simulink model "AMPC_CSimOldNN_genLinearModelBased"  (R2019b)
settings: Solver=FixedStepAuto  StartTime=0.0  StopTime=Time(end)  FixedStep=Time(2)  RelTol=1e-3
libraries: neural x31, mpclib x1, cstblocks x1
settings Model: Creator=Shouvik Chakraborty  LastModifiedBy=shouv
settings SFSimCC: CustomCodeUndefinedFunction=UseInterfaceOnly

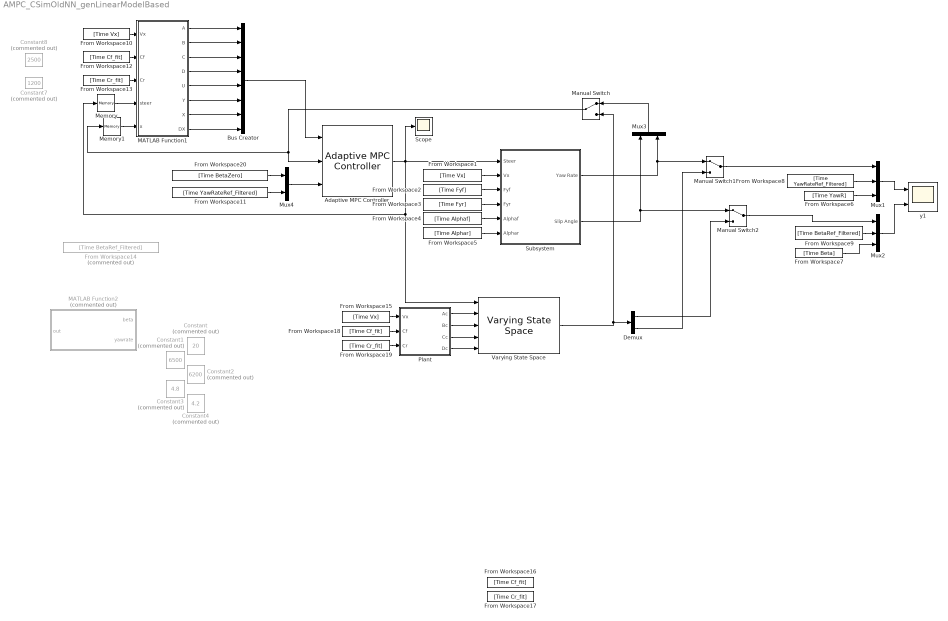
== system AMPC_CSimOldNN_genLinearModelBased ==
  Adaptive MPC Controller : mpclib/Adaptive MPC Controller  SCDEnableBlockLinearizationSpecification=on  mpcobj=adaptivempc1  enable_value=0  updateMPCinCallerWorkspace=on  md_inport=off  mv_inport=off  uref_inport=off  return_cost=off  return_mvseq=off  return_qpstatus=off  return_xseq=off  return_state=off  return_ovseq=off  state_inport=off  isltv_plant=off  umin_inport=off  umax_inport=off  ymin_inport=off  ymax_inport=off  cc_inport=off  ywt_inport=off  uwt_inport=off  duwt_inport=off  rhoeps_inport=off  pm_inport=off  MaximumP=10  HorizonChoice=FixedHorizon  BlockDataType=double  SampleTimeInherited=off  switch_inport=off
      settings: SourceProductName=Model Predictive Control Toolbox
  Bus Creator : BusCreator  Inputs=8
  Constant : Constant  Commented=on  Value=20
  Constant1 : Constant  Commented=on  Value=6500
  Constant2 : Constant  Commented=on  Value=6200
  Constant3 : Constant  Commented=on  Value=4.8
  Constant4 : Constant  Commented=on  Value=4.2
  Constant7 : Constant  Commented=on  Value=1200
  Constant8 : Constant  Commented=on  Value=2500
  Demux : Demux  Outputs=2
  From Workspace1 : FromWorkspace  VariableName=[Time Vx]  SampleTime=0
  From Workspace10 : FromWorkspace  VariableName=[Time Vx]  SampleTime=0
  From Workspace11 : FromWorkspace  VariableName=[Time YawRateRef_Filtered]  SampleTime=0
  From Workspace12 : FromWorkspace  VariableName=[Time Cf_fit]  SampleTime=0
  From Workspace13 : FromWorkspace  VariableName=[Time Cr_fit]  SampleTime=0
  From Workspace14 : FromWorkspace  Commented=on  VariableName=[Time BetaRef_Filtered]  SampleTime=0
  From Workspace15 : FromWorkspace  VariableName=[Time Vx]  SampleTime=0
  From Workspace16 : FromWorkspace  VariableName=[Time Cf_fit]  SampleTime=0
  From Workspace17 : FromWorkspace  VariableName=[Time Cr_fit]  SampleTime=0
  From Workspace18 : FromWorkspace  VariableName=[Time Cf_fit]  SampleTime=0
  From Workspace19 : FromWorkspace  VariableName=[Time Cr_fit]  SampleTime=0
  From Workspace2 : FromWorkspace  VariableName=[Time Fyf]  SampleTime=0
  From Workspace20 : FromWorkspace  VariableName=[Time BetaZero]  SampleTime=0
  From Workspace3 : FromWorkspace  VariableName=[Time Fyr]  SampleTime=0
  From Workspace4 : FromWorkspace  VariableName=[Time Alphaf]  SampleTime=0
  From Workspace5 : FromWorkspace  VariableName=[Time Alphar]  SampleTime=0
  From Workspace6 : FromWorkspace  VariableName=[Time YawR]  SampleTime=0
  From Workspace7 : FromWorkspace  VariableName=[Time Beta]  SampleTime=0
  From Workspace8 : FromWorkspace  VariableName=[Time YawRateRef_Filtered]  SampleTime=0
  From Workspace9 : FromWorkspace  VariableName=[Time BetaRef_Filtered]  SampleTime=0
  MATLAB Function1 : MATLAB Function  TreatAsAtomicUnit=on
  MATLAB Function2 : MATLAB Function  Commented=on  TreatAsAtomicUnit=on
  Manual Switch : ManualSwitch
  Manual Switch1 : ManualSwitch
  Manual Switch2 : ManualSwitch
  Memory : Memory
  Memory1 : Memory
  Mux1 : Mux  Inputs=3
  Mux2 : Mux  Inputs=3
  Mux3 : Mux  Inputs=2
  Mux4 : Mux  Inputs=2
  Plant : MATLAB Function  TreatAsAtomicUnit=on
  Scope : Scope
  Subsystem : Subsystem
  Varying State Space : cstblocks/Linear Parameter Varying/Varying State Space  x0=0  xNames=''  OutputX=off  OutputDX=off
      settings: SourceProductName=Control System Toolbox
  y1 : Scope  NumInputPorts=2
      mask Display: e = 0.06;c1 = [120 230 180]/255;c2 = ([120 230 180]+0)/(256+128);c3 = ([120 230 180]+128)/(256+128);patch([0 1 1 0],[0 0 1 1],c1);patch([0 1 1 1-e 1-e 0+e],[0 0 1 1-e 0+e 0+e],c2);patch([0 0 1 1-e 0+e 0+e],[0 1 1 1-e 1-e 0+e],c3);plot([0 1 1 0 0],[0 0 1 1 0]);plot([0.15 0.85 0.85 0.15 0.15],[0.5 0.5 0.85 0.85 0.5]);
  wires:
  From Workspace7/1 -> Mux2/3
  Mux2/1 -> y1/2
  MATLAB Function1/3(C) -> Bus Creator/3
  MATLAB Function1/5(U) -> Bus Creator/5
  MATLAB Function1/4(D) -> Bus Creator/4
  Mux1/1 -> y1/1
  MATLAB Function1/6(Y) -> Bus Creator/6
  From Workspace11/1 -> Mux4/2
  Subsystem/1(Yaw Rate) -> Mux3/2, Manual Switch1/1
  MATLAB Function1/2(B) -> Bus Creator/2
  Subsystem/2(Slip Angle) -> Manual Switch2/1, Mux3/1
  From Workspace9/1 -> Mux2/2
  MATLAB Function1/1(A) -> Bus Creator/1
  Mux4/1 -> Adaptive MPC Controller/3
  From Workspace1/1 -> Subsystem/2(Vx)
  MATLAB Function1/7(X) -> Bus Creator/7
  Memory/1 -> MATLAB Function1/4(steer)
  MATLAB Function1/8(DX) -> Bus Creator/8
  Bus Creator/1 -> Adaptive MPC Controller/1
  From Workspace5/1 -> Subsystem/6(Alphar)
  From Workspace20/1 -> Mux4/1
  From Workspace6/1 -> Mux1/3
  From Workspace3/1 -> Subsystem/4(Fyr)
  From Workspace12/1 -> MATLAB Function1/2(Cf)
  From Workspace10/1 -> MATLAB Function1/1(Vx)
  From Workspace13/1 -> MATLAB Function1/3(Cr)
  From Workspace8/1 -> Mux1/2
  Manual Switch/1 -> Memory1/1, Adaptive MPC Controller/2
  From Workspace2/1 -> Subsystem/3(Fyf)
  From Workspace4/1 -> Subsystem/5(Alphaf)
  From Workspace15/1 -> Plant/1(Vx)
  From Workspace18/1 -> Plant/2(Cf)
  From Workspace19/1 -> Plant/3(Cr)
  Adaptive MPC Controller/1 -> Varying State Space/1, Memory/1, Subsystem/1(Steer), Scope/1
  Mux3/1 -> Manual Switch/1
  Manual Switch1/1 -> Mux1/1
  Varying State Space/1 -> Demux/1, Manual Switch/2
  Manual Switch2/1 -> Mux2/1
  Demux/1 -> Manual Switch2/2
  Demux/2 -> Manual Switch1/2
  Plant/1(Ac) -> Varying State Space/2
  Plant/2(Bc) -> Varying State Space/3
  Plant/3(Cc) -> Varying State Space/4
  Plant/4(Dc) -> Varying State Space/5
  Memory1/1 -> MATLAB Function1/5(x)

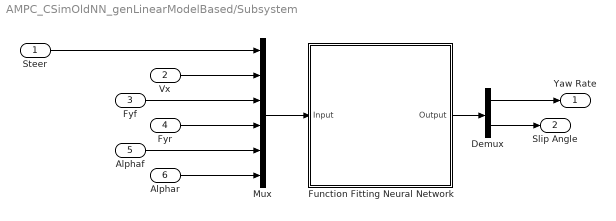
== system AMPC_CSimOldNN_genLinearModelBased/Subsystem ==
  Steer : Inport
  Vx : Inport  Port=2
  Fyf : Inport  Port=3
  Fyr : Inport  Port=4
  Alphaf : Inport  Port=5
  Alphar : Inport  Port=6
  Demux : Demux  Outputs=2
  Function Fitting Neural Network : Subsystem
      mask help: Function Fitting Neural Network
      mask Display: e = 0.06;c1 = [120 150 230]/255;c2 = ([120 150 230]+0)/383;c3 = ([120 150 230]+128)/383;patch([0 1 1 0],[0 0 1 1],c1);patch([0 1 1 1-e 1-e 0+e],[0 0 1 1-e 0+e 0+e],c2);patch([0 0 1 1-e 0+e 0+e],[0 1 1 1-e 1-e 0+e],c3);plot([0 1 1 0 0],[0 0 1 1 0]);fprintf('NNET');port_label('input',1,' Input');port_label('output',1,'Output ');
  Mux : Mux  Inputs=6
  Yaw Rate : Outport  VectorParamsAs1DForOutWhenUnconnected=off
  Slip Angle : Outport  Port=2  VectorParamsAs1DForOutWhenUnconnected=off
  wires:
  Vx/1 -> Mux/2
  Fyr/1 -> Mux/4
  Mux/1 -> Function Fitting Neural Network/1(Input)
  Steer/1 -> Mux/1
  Function Fitting Neural Network/1(Output) -> Demux/1
  Demux/2 -> Slip Angle/1
  Fyf/1 -> Mux/3
  Alphaf/1 -> Mux/5
  Demux/1 -> Yaw Rate/1
  Alphar/1 -> Mux/6

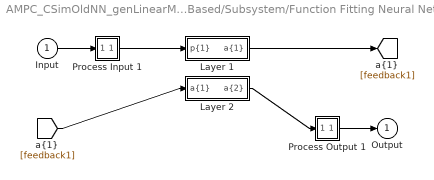
== system AMPC_CSimOldNN_genLinearModelBased/Subsystem/Function Fitting Neural Network ==
  Input : Inport  PortDimensions=6
      mask Display: e = 0.06;c1 = [120 230 180]/255;c2 = ([120 230 180]+0)/(256+128);c3 = ([120 230 180]+128)/(256+128);patch([0 1 1 0],[0 0 1 1],c1);patch([0 1 1 1-e 1-e 0+e],[0 0 1 1-e 0+e 0+e],c2);patch([0 0 1 1-e 0+e 0+e],[0 1 1 1-e 1-e 0+e],c3);plot([0 1 1 0 0],[0 0 1 1 0]);
  Layer 1 : Subsystem
      mask Display: e = 0.06;c1 = [120 150 230]/255;c2 = ([120 150 230]+0)/383;c3 = ([120 150 230]+128)/383;patch([0 1 1 0],[0 0 1 1],c1);patch([0 1 1 1-e 1-e 0+e],[0 0 1 1-e 0+e 0+e],c2);patch([0 0 1 1-e 0+e 0+e],[0 1 1 1-e 1-e 0+e],c3);plot([0 1 1 0 0],[0 0 1 1 0]);
  Layer 2 : Subsystem
      mask Display: e = 0.06;c1 = [120 150 230]/255;c2 = ([120 150 230]+0)/383;c3 = ([120 150 230]+128)/383;patch([0 1 1 0],[0 0 1 1],c1);patch([0 1 1 1-e 1-e 0+e],[0 0 1 1-e 0+e 0+e],c2);patch([0 0 1 1-e 0+e 0+e],[0 1 1 1-e 1-e 0+e],c3);plot([0 1 1 0 0],[0 0 1 1 0]);
  Process Input 1 : Subsystem
      mask Display: e = 0.06;c1 = [120 150 230]/255;c2 = ([120 150 230]+0)/383;c3 = ([120 150 230]+128)/383;patch([0 1 1 0],[0 0 1 1],c1);patch([0 1 1 1-e 1-e 0+e],[0 0 1 1-e 0+e 0+e],c2);patch([0 0 1 1-e 0+e 0+e],[0 1 1 1-e 1-e 0+e],c3);plot([0 1 1 0 0],[0 0 1 1 0]);
  Process Output 1 : Subsystem
      mask Display: e = 0.06;c1 = [120 150 230]/255;c2 = ([120 150 230]+0)/383;c3 = ([120 150 230]+128)/383;patch([0 1 1 0],[0 0 1 1],c1);patch([0 1 1 1-e 1-e 0+e],[0 0 1 1-e 0+e 0+e],c2);patch([0 0 1 1-e 0+e 0+e],[0 1 1 1-e 1-e 0+e],c3);plot([0 1 1 0 0],[0 0 1 1 0]);
  Output : Outport  InitialOutput=[0;0]  VectorParamsAs1DForOutWhenUnconnected=off
      mask Display: e = 0.06;c1 = [120 230 180]/255;c2 = ([120 230 180]+0)/(256+128);c3 = ([120 230 180]+128)/(256+128);patch([0 1 1 0],[0 0 1 1],c1);patch([0 1 1 1-e 1-e 0+e],[0 0 1 1-e 0+e 0+e],c2);patch([0 0 1 1-e 0+e 0+e],[0 1 1 1-e 1-e 0+e],c3);plot([0 1 1 0 0],[0 0 1 1 0]);
  wires:
  Input/1 -> Process Input 1/1(x)
  Process Output 1/1(y) -> Output/1
  Process Input 1/1(p) -> Layer 1/1("p{1}")
  Layer 1/1("a{1}") -> [feedback1]
  [feedback1] -> Layer 2/1("a{1} ")
  Layer 2/1("a{2}") -> Process Output 1/1(a)

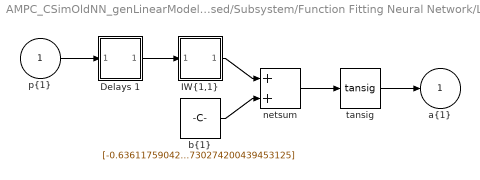
== system AMPC_CSimOldNN_genLinearModelBased/Subsystem/Function Fitting Neural Network/Layer 1 ==
  "p{1}" : Inport  PortDimensions=6
      mask Display: e = 0.06;c1 = [120 230 180]/255;c2 = ([120 230 180]+0)/(256+128);c3 = ([120 230 180]+128)/(256+128);patch([0 1 1 0],[0 0 1 1],c1);patch([0 1 1 1-e 1-e 0+e],[0 0 1 1-e 0+e 0+e],c2);patch([0 0 1 1-e 0+e 0+e],[0 1 1 1-e 1-e 0+e],c3);plot([0 1 1 0 0],[0 0 1 1 0]);
  Delays 1 : Subsystem
      mask Display: e = 0.06;c1 = [120 150 230]/255;c2 = ([120 150 230]+0)/383;c3 = ([120 150 230]+128)/383;patch([0 1 1 0],[0 0 1 1],c1);patch([0 1 1 1-e 1-e 0+e],[0 0 1 1-e 0+e 0+e],c2);patch([0 0 1 1-e 0+e 0+e],[0 1 1 1-e 1-e 0+e],c3);plot([0 1 1 0 0],[0 0 1 1 0]);disp('0');
  "IW{1,1}" : Subsystem
      mask Display: e = 0.06;c1 = [120 150 230]/255;c2 = ([120 150 230]+0)/383;c3 = ([120 150 230]+128)/383;patch([0 1 1 0],[0 0 1 1],c1);patch([0 1 1 1-e 1-e 0+e],[0 0 1 1-e 0+e 0+e],c2);patch([0 0 1 1-e 0+e 0+e],[0 1 1 1-e 1-e 0+e],c3);plot([0 1 1 0 0],[0 0 1 1 0]);disp('W');
  "b{1}" : Constant  Value=[-0.63611759042286653009767860567080788314342498779296875;0.0678442132315502932637940602944581769406795501708984375;0.920857296622486831694232023437507450580596923828125;0.3400400984533717974045430310070514678955078125;1.068840554455138036615835517295636236667633056640625;-1.1840912053117917945854742356459610164165496826171875;2.1641288663140425541087097371928393840789794921875;-0.0026747980112842586163102165386362685239873826503753662109375;-1.2400348389807971383191897984943352639675140380859375;0.05422832279501725583070737002344685606658458709716796875;1.090956117788687063097086138441227376461029052734375;-0.538161801971245079556638302165083587169647216796875;-0.0971368234755809190072994852016563527286052703857421875;-0.65424405420957143508786657548625953495502471923828125;-0.0294578949609712141544104468948717112652957439422607421875;-0.055152953134630144926831007978762499988079071044921875;1.1922936756190452012305058815400116145610809326171875;-0.4982569158340737214274440702865831553936004638671875;1.4572737748217508002568365554907359182834625244140625;-0.71536140771868428345214852015487849712371826171875;0.121920011275389150728898357556317932903766632080078125;-0.08237235483539008529252356538563617505133152008056640625;0.0065354555755173411590863707942844484932720661163330078125;0.57411081788391593594411688172840513288974761962890625;0.890585538278589883276481486973352730274200439453125]
      mask Display: e = 0.06;c1 = [120 150 230]/255;c2 = ([120 150 230]+0)/383;c3 = ([120 150 230]+128)/383;patch([0 1 1 0],[0 0 1 1],c1);patch([0 1 1 1-e 1-e 0+e],[0 0 1 1-e 0+e 0+e],c2);patch([0 0 1 1-e 0+e 0+e],[0 1 1 1-e 1-e 0+e],c3);plot([0 1 1 0 0],[0 0 1 1 0]);disp('b');
  netsum : Sum  Inputs=2  SaturateOnIntegerOverflow=on  InputSameDT=on  OutDataTypeStr=Inherit: Same as first input
      mask Display: e = 0.06;c1 = [120 150 230]/255;c2 = ([120 150 230]+0)/383;c3 = ([120 150 230]+128)/383;patch([0 1 1 0],[0 0 1 1],c1);patch([0 1 1 1-e 1-e 0+e],[0 0 1 1-e 0+e 0+e],c2);patch([0 0 1 1-e 0+e 0+e],[0 1 1 1-e 1-e 0+e],c3);plot([0 1 1 0 0],[0 0 1 1 0]);disp('+');
  tansig : neural/Transfer Functions/tansig
      settings: SourceProductName=MATLAB Runtime - Deep Learning Toolbox  SourceProductBaseCode=Missing
  "a{1}" : Outport  InitialOutput=[0;0;0;0;0;0;0;0;0;0;0;0;0;0;0;0;0;0;0;0;0;0;0;0;0]  VectorParamsAs1DForOutWhenUnconnected=off
      mask Display: e = 0.06;c1 = [120 230 180]/255;c2 = ([120 230 180]+0)/(256+128);c3 = ([120 230 180]+128)/(256+128);patch([0 1 1 0],[0 0 1 1],c1);patch([0 1 1 1-e 1-e 0+e],[0 0 1 1-e 0+e 0+e],c2);patch([0 0 1 1-e 0+e 0+e],[0 1 1 1-e 1-e 0+e],c3);plot([0 1 1 0 0],[0 0 1 1 0]);
  wires:
  "p{1}"/1 -> Delays 1/1("p{1}")
  Delays 1/1("pd{1,1}") -> "IW{1,1}"/1("pd{1,1}")
  "IW{1,1}"/1("iz{1,1}") -> netsum/1
  "b{1}"/1 -> netsum/2
  netsum/1 -> tansig/1
  tansig/1 -> "a{1}"/1

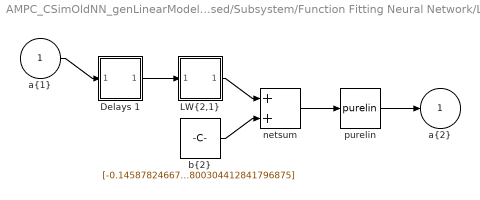
== system AMPC_CSimOldNN_genLinearModelBased/Subsystem/Function Fitting Neural Network/Layer 2 ==
  "a{1} " : Inport  PortDimensions=25
      mask Display: e = 0.06;c1 = [120 230 180]/255;c2 = ([120 230 180]+0)/(256+128);c3 = ([120 230 180]+128)/(256+128);patch([0 1 1 0],[0 0 1 1],c1);patch([0 1 1 1-e 1-e 0+e],[0 0 1 1-e 0+e 0+e],c2);patch([0 0 1 1-e 0+e 0+e],[0 1 1 1-e 1-e 0+e],c3);plot([0 1 1 0 0],[0 0 1 1 0]);
  Delays 1 : Subsystem
      mask Display: e = 0.06;c1 = [120 150 230]/255;c2 = ([120 150 230]+0)/383;c3 = ([120 150 230]+128)/383;patch([0 1 1 0],[0 0 1 1],c1);patch([0 1 1 1-e 1-e 0+e],[0 0 1 1-e 0+e 0+e],c2);patch([0 0 1 1-e 0+e 0+e],[0 1 1 1-e 1-e 0+e],c3);plot([0 1 1 0 0],[0 0 1 1 0]);disp('0');
  "LW{2,1}" : Subsystem
      mask Display: e = 0.06;c1 = [120 150 230]/255;c2 = ([120 150 230]+0)/383;c3 = ([120 150 230]+128)/383;patch([0 1 1 0],[0 0 1 1],c1);patch([0 1 1 1-e 1-e 0+e],[0 0 1 1-e 0+e 0+e],c2);patch([0 0 1 1-e 0+e 0+e],[0 1 1 1-e 1-e 0+e],c3);plot([0 1 1 0 0],[0 0 1 1 0]);disp('W');
  "b{2}" : Constant  Value=[-0.1458782466754957596322128665633499622344970703125;0.36038774408484908207128682988695800304412841796875]
      mask Display: e = 0.06;c1 = [120 150 230]/255;c2 = ([120 150 230]+0)/383;c3 = ([120 150 230]+128)/383;patch([0 1 1 0],[0 0 1 1],c1);patch([0 1 1 1-e 1-e 0+e],[0 0 1 1-e 0+e 0+e],c2);patch([0 0 1 1-e 0+e 0+e],[0 1 1 1-e 1-e 0+e],c3);plot([0 1 1 0 0],[0 0 1 1 0]);disp('b');
  netsum : Sum  Inputs=2  SaturateOnIntegerOverflow=on  InputSameDT=on  OutDataTypeStr=Inherit: Same as first input
      mask Display: e = 0.06;c1 = [120 150 230]/255;c2 = ([120 150 230]+0)/383;c3 = ([120 150 230]+128)/383;patch([0 1 1 0],[0 0 1 1],c1);patch([0 1 1 1-e 1-e 0+e],[0 0 1 1-e 0+e 0+e],c2);patch([0 0 1 1-e 0+e 0+e],[0 1 1 1-e 1-e 0+e],c3);plot([0 1 1 0 0],[0 0 1 1 0]);disp('+');
  purelin : neural/Transfer Functions/purelin
      settings: SourceProductName=MATLAB Runtime - Deep Learning Toolbox  SourceProductBaseCode=Missing
  "a{2}" : Outport  InitialOutput=[0;0]  VectorParamsAs1DForOutWhenUnconnected=off
      mask Display: e = 0.06;c1 = [120 230 180]/255;c2 = ([120 230 180]+0)/(256+128);c3 = ([120 230 180]+128)/(256+128);patch([0 1 1 0],[0 0 1 1],c1);patch([0 1 1 1-e 1-e 0+e],[0 0 1 1-e 0+e 0+e],c2);patch([0 0 1 1-e 0+e 0+e],[0 1 1 1-e 1-e 0+e],c3);plot([0 1 1 0 0],[0 0 1 1 0]);
  wires:
  "a{1} "/1 -> Delays 1/1("p{2}")
  Delays 1/1("pd{2,1}") -> "LW{2,1}"/1("ad{2,1}")
  "LW{2,1}"/1("lz{2,1}") -> netsum/1
  "b{2}"/1 -> netsum/2
  netsum/1 -> purelin/1
  purelin/1 -> "a{2}"/1

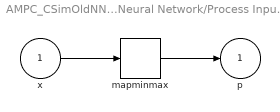
== system AMPC_CSimOldNN_genLinearModelBased/Subsystem/Function Fitting Neural Network/Process Input 1 ==
  x : Inport  PortDimensions=6
      mask Display: e = 0.06;c1 = [120 230 180]/255;c2 = ([120 230 180]+0)/(256+128);c3 = ([120 230 180]+128)/(256+128);patch([0 1 1 0],[0 0 1 1],c1);patch([0 1 1 1-e 1-e 0+e],[0 0 1 1-e 0+e 0+e],c2);patch([0 0 1 1-e 0+e 0+e],[0 1 1 1-e 1-e 0+e],c3);plot([0 1 1 0 0],[0 0 1 1 0]);
  mapminmax : neural/Processing Functions/mapminmax  xmin=[-0.736012004800314478814016183605;16.1847326490614165095394128002;-8474.6336669921875;-6221.221435546875;-33.8465023040771484375;-5.6262662410736083984375]  xmax=[0.5937319910620723062422143812;17.1756839752197265625;8619.833984375;7007.822021484375;42.2919864654541015625;5.51491069793701171875]  ymin=-1  ymax=1
      settings: SourceProductName=MATLAB Runtime - Deep Learning Toolbox  SourceProductBaseCode=Missing
  p : Outport  PortDimensions=6  VectorParamsAs1DForOutWhenUnconnected=off
      mask Display: e = 0.06;c1 = [120 230 180]/255;c2 = ([120 230 180]+0)/(256+128);c3 = ([120 230 180]+128)/(256+128);patch([0 1 1 0],[0 0 1 1],c1);patch([0 1 1 1-e 1-e 0+e],[0 0 1 1-e 0+e 0+e],c2);patch([0 0 1 1-e 0+e 0+e],[0 1 1 1-e 1-e 0+e],c3);plot([0 1 1 0 0],[0 0 1 1 0]);
  wires:
  x/1 -> mapminmax/1
  mapminmax/1 -> p/1

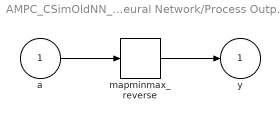
== system AMPC_CSimOldNN_genLinearModelBased/Subsystem/Function Fitting Neural Network/Process Output 1 ==
  a : Inport  PortDimensions=2
      mask Display: e = 0.06;c1 = [120 230 180]/255;c2 = ([120 230 180]+0)/(256+128);c3 = ([120 230 180]+128)/(256+128);patch([0 1 1 0],[0 0 1 1],c1);patch([0 1 1 1-e 1-e 0+e],[0 0 1 1-e 0+e 0+e],c2);patch([0 0 1 1-e 0+e 0+e],[0 1 1 1-e 1-e 0+e],c3);plot([0 1 1 0 0],[0 0 1 1 0]);
  mapminmax_reverse : neural/Processing Functions/mapminmax_reverse  xmin=[-0.543732972519084034601632993144;-0.0494721578943973228081887327789]  xmax=[0.555606642949688755983572718833;0.0398466573158211059824118649431]  ymin=-1  ymax=1
      settings: SourceProductName=MATLAB Runtime - Deep Learning Toolbox  SourceProductBaseCode=Missing
  y : Outport  PortDimensions=2  VectorParamsAs1DForOutWhenUnconnected=off
      mask Display: e = 0.06;c1 = [120 230 180]/255;c2 = ([120 230 180]+0)/(256+128);c3 = ([120 230 180]+128)/(256+128);patch([0 1 1 0],[0 0 1 1],c1);patch([0 1 1 1-e 1-e 0+e],[0 0 1 1-e 0+e 0+e],c2);patch([0 0 1 1-e 0+e 0+e],[0 1 1 1-e 1-e 0+e],c3);plot([0 1 1 0 0],[0 0 1 1 0]);
  wires:
  a/1 -> mapminmax_reverse/1
  mapminmax_reverse/1 -> y/1

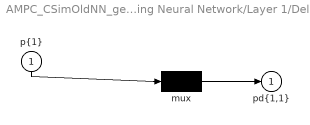
== system AMPC_CSimOldNN_genLinearModelBased/Subsystem/Function Fitting Neural Network/Layer 1/Delays 1 ==
  "p{1}" : Inport  PortDimensions=6
      mask Display: e = 0.06;c1 = [120 230 180]/255;c2 = ([120 230 180]+0)/(256+128);c3 = ([120 230 180]+128)/(256+128);patch([0 1 1 0],[0 0 1 1],c1);patch([0 1 1 1-e 1-e 0+e],[0 0 1 1-e 0+e 0+e],c2);patch([0 0 1 1-e 0+e 0+e],[0 1 1 1-e 1-e 0+e],c3);plot([0 1 1 0 0],[0 0 1 1 0]);
  mux : Mux  Inputs=1
      mask Display: e = 0.06;c1 = [120 150 230]/255;c2 = ([120 150 230]+0)/383;c3 = ([120 150 230]+128)/383;patch([0 1 1 0],[0 0 1 1],c1);patch([0 1 1 1-e 1-e 0+e],[0 0 1 1-e 0+e 0+e],c2);patch([0 0 1 1-e 0+e 0+e],[0 1 1 1-e 1-e 0+e],c3);plot([0 1 1 0 0],[0 0 1 1 0]);disp('Mux')
  "pd{1,1}" : Outport  VectorParamsAs1DForOutWhenUnconnected=off
      mask Display: e = 0.06;c1 = [120 230 180]/255;c2 = ([120 230 180]+0)/(256+128);c3 = ([120 230 180]+128)/(256+128);patch([0 1 1 0],[0 0 1 1],c1);patch([0 1 1 1-e 1-e 0+e],[0 0 1 1-e 0+e 0+e],c2);patch([0 0 1 1-e 0+e 0+e],[0 1 1 1-e 1-e 0+e],c3);plot([0 1 1 0 0],[0 0 1 1 0]);
  wires:
  "p{1}"/1 -> mux/1
  mux/1 -> "pd{1,1}"/1

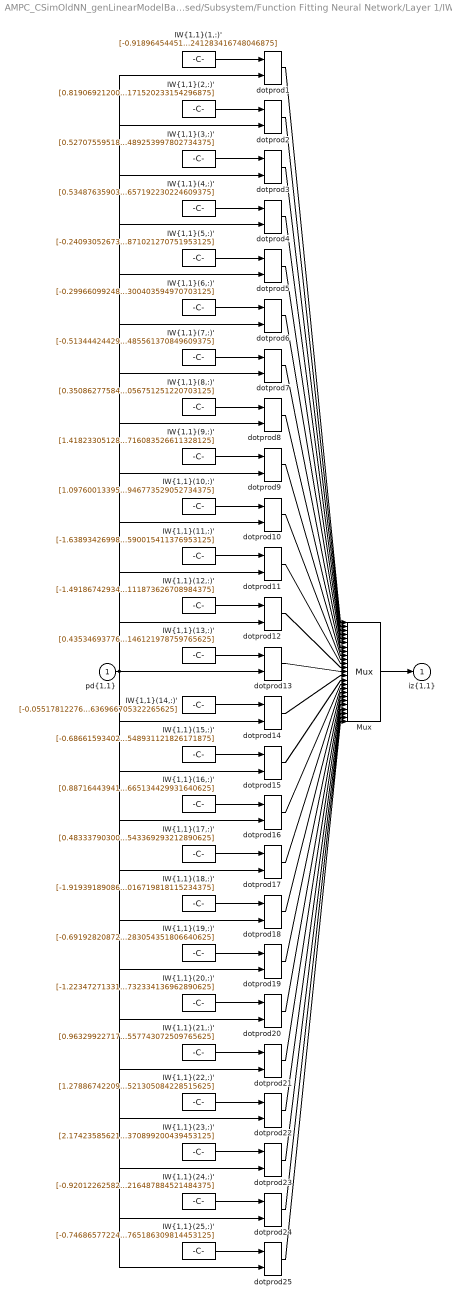
== system AMPC_CSimOldNN_genLinearModelBased/Subsystem/Function Fitting Neural Network/Layer 1/IW{1,1} ==
  "pd{1,1}" : Inport  PortDimensions=6
      mask Display: e = 0.06;c1 = [120 230 180]/255;c2 = ([120 230 180]+0)/(256+128);c3 = ([120 230 180]+128)/(256+128);patch([0 1 1 0],[0 0 1 1],c1);patch([0 1 1 1-e 1-e 0+e],[0 0 1 1-e 0+e 0+e],c2);patch([0 0 1 1-e 0+e 0+e],[0 1 1 1-e 1-e 0+e],c3);plot([0 1 1 0 0],[0 0 1 1 0]);
  "IW{1,1}(1,:)'" : Constant  Value=[-0.91896454451869669100005921791307628154754638671875;2.807406064374065923772150199511088430881500244140625;-0.32650530029088009609239406927372328937053680419921875;-0.68212399974366133559300351407728157937526702880859375;0.55443567787012237868538022667053155601024627685546875;-0.328157572076140435779478821132215671241283416748046875]
      mask Display: e = 0.06;c1 = [120 150 230]/255;c2 = ([120 150 230]+0)/383;c3 = ([120 150 230]+128)/383;patch([0 1 1 0],[0 0 1 1],c1);patch([0 1 1 1-e 1-e 0+e],[0 0 1 1-e 0+e 0+e],c2);patch([0 0 1 1-e 0+e 0+e],[0 1 1 1-e 1-e 0+e],c3);plot([0 1 1 0 0],[0 0 1 1 0]);disp('Weights');
  "IW{1,1}(10,:)'" : Constant  Value=[1.097600133959441226494391230517067015171051025390625;-0.07827061444567622039425458524419809691607952117919921875;-0.38990454765808413295502532491809688508510589599609375;0.46998928551050112023546034833998419344425201416015625;0.4354289920842753236485123125021345913410186767578125;-0.59819487501920798333543416447355411946773529052734375]
      mask Display: e = 0.06;c1 = [120 150 230]/255;c2 = ([120 150 230]+0)/383;c3 = ([120 150 230]+128)/383;patch([0 1 1 0],[0 0 1 1],c1);patch([0 1 1 1-e 1-e 0+e],[0 0 1 1-e 0+e 0+e],c2);patch([0 0 1 1-e 0+e 0+e],[0 1 1 1-e 1-e 0+e],c3);plot([0 1 1 0 0],[0 0 1 1 0]);disp('Weights');
  "IW{1,1}(11,:)'" : Constant  Value=[-1.6389342699858098217902124815736897289752960205078125;-0.7309100789032456635396783894975669682025909423828125;0.0018010659112654837758771275701974445837549865245819091796875;0.83129641458116487751084378032828681170940399169921875;-0.93893409236719238553092736765393055975437164306640625;0.084419703238978460735353337440756149590015411376953125]
      mask Display: e = 0.06;c1 = [120 150 230]/255;c2 = ([120 150 230]+0)/383;c3 = ([120 150 230]+128)/383;patch([0 1 1 0],[0 0 1 1],c1);patch([0 1 1 1-e 1-e 0+e],[0 0 1 1-e 0+e 0+e],c2);patch([0 0 1 1-e 0+e 0+e],[0 1 1 1-e 1-e 0+e],c3);plot([0 1 1 0 0],[0 0 1 1 0]);disp('Weights');
  "IW{1,1}(12,:)'" : Constant  Value=[-1.4918674293447633516507266904227435588836669921875;0.52049473620865904788246325551881454885005950927734375;-0.272842583889991330270419211956323124468326568603515625;-0.5921939615822207070294780351105146110057830810546875;-1.6000734146301442972770701089757494628429412841796875;-0.7163345210483613723084772573201917111873626708984375]
      mask Display: e = 0.06;c1 = [120 150 230]/255;c2 = ([120 150 230]+0)/383;c3 = ([120 150 230]+128)/383;patch([0 1 1 0],[0 0 1 1],c1);patch([0 1 1 1-e 1-e 0+e],[0 0 1 1-e 0+e 0+e],c2);patch([0 0 1 1-e 0+e 0+e],[0 1 1 1-e 1-e 0+e],c3);plot([0 1 1 0 0],[0 0 1 1 0]);disp('Weights');
  "IW{1,1}(13,:)'" : Constant  Value=[0.4353469377680905250116438764962367713451385498046875;-0.84085297783017975969954704851261340081691741943359375;-0.3262431999570882812378158632782287895679473876953125;-0.03343748267568195930987684505453216843307018280029296875;0.7569219535729778680632762188906781375408172607421875;-0.336770011411867520312313217800692655146121978759765625]
      mask Display: e = 0.06;c1 = [120 150 230]/255;c2 = ([120 150 230]+0)/383;c3 = ([120 150 230]+128)/383;patch([0 1 1 0],[0 0 1 1],c1);patch([0 1 1 1-e 1-e 0+e],[0 0 1 1-e 0+e 0+e],c2);patch([0 0 1 1-e 0+e 0+e],[0 1 1 1-e 1-e 0+e],c3);plot([0 1 1 0 0],[0 0 1 1 0]);disp('Weights');
  "IW{1,1}(14,:)'" : Constant  Value=[-0.055178122760997337648003480126135400496423244476318359375;-1.4381626335296340268854464738979004323482513427734375;0.1875648565884424356919879528504679910838603973388671875;-0.53640519002087516664545319144963286817073822021484375;-1.0068525371299339443709186525666154921054840087890625;0.160847593541183275789308027015067636966705322265625]
      mask Display: e = 0.06;c1 = [120 150 230]/255;c2 = ([120 150 230]+0)/383;c3 = ([120 150 230]+128)/383;patch([0 1 1 0],[0 0 1 1],c1);patch([0 1 1 1-e 1-e 0+e],[0 0 1 1-e 0+e 0+e],c2);patch([0 0 1 1-e 0+e 0+e],[0 1 1 1-e 1-e 0+e],c3);plot([0 1 1 0 0],[0 0 1 1 0]);disp('Weights');
  "IW{1,1}(15,:)'" : Constant  Value=[-0.686615934023023566368237879942171275615692138671875;0.426894044409089457037254078386467881500720977783203125;-0.60810228251544184985277752275578677654266357421875;0.1522748062778661870542151746121817268431186676025390625;-2.1099858845401460172297447570599615573883056640625;0.1713882654697056195924886878856341354548931121826171875]
      mask Display: e = 0.06;c1 = [120 150 230]/255;c2 = ([120 150 230]+0)/383;c3 = ([120 150 230]+128)/383;patch([0 1 1 0],[0 0 1 1],c1);patch([0 1 1 1-e 1-e 0+e],[0 0 1 1-e 0+e 0+e],c2);patch([0 0 1 1-e 0+e 0+e],[0 1 1 1-e 1-e 0+e],c3);plot([0 1 1 0 0],[0 0 1 1 0]);disp('Weights');
  "IW{1,1}(16,:)'" : Constant  Value=[0.88716443941147471452524086998892016708850860595703125;0.40313159970102241391742836640332825481891632080078125;-0.015657524645655340744809791431180201470851898193359375;-0.478263451738349443242981351431808434426784515380859375;0.3859891211729997717583273697528056800365447998046875;0.6315189817233604063773100278922356665134429931640625]
      mask Display: e = 0.06;c1 = [120 150 230]/255;c2 = ([120 150 230]+0)/383;c3 = ([120 150 230]+128)/383;patch([0 1 1 0],[0 0 1 1],c1);patch([0 1 1 1-e 1-e 0+e],[0 0 1 1-e 0+e 0+e],c2);patch([0 0 1 1-e 0+e 0+e],[0 1 1 1-e 1-e 0+e],c3);plot([0 1 1 0 0],[0 0 1 1 0]);disp('Weights');
  "IW{1,1}(17,:)'" : Constant  Value=[0.48333790300379242399486656722729094326496124267578125;0.0251588125096972210770207567520628799684345722198486328125;-0.67153040371300332100901187004637904465198516845703125;0.46244925298389250034603037420311011373996734619140625;-0.126361383991284270678079337812960147857666015625;-0.9536652713805617853637386360787786543369293212890625]
      mask Display: e = 0.06;c1 = [120 150 230]/255;c2 = ([120 150 230]+0)/383;c3 = ([120 150 230]+128)/383;patch([0 1 1 0],[0 0 1 1],c1);patch([0 1 1 1-e 1-e 0+e],[0 0 1 1-e 0+e 0+e],c2);patch([0 0 1 1-e 0+e 0+e],[0 1 1 1-e 1-e 0+e],c3);plot([0 1 1 0 0],[0 0 1 1 0]);disp('Weights');
  "IW{1,1}(18,:)'" : Constant  Value=[-1.919391890863494598562510873307473957538604736328125;2.760761832853932506992578055360354483127593994140625;0.166517652488541612054717688806704245507717132568359375;0.554430338119628718374087839038111269474029541015625;0.9634316882260487435729601202183403074741363525390625;-1.5238850536123587087189434896572493016719818115234375]
      mask Display: e = 0.06;c1 = [120 150 230]/255;c2 = ([120 150 230]+0)/383;c3 = ([120 150 230]+128)/383;patch([0 1 1 0],[0 0 1 1],c1);patch([0 1 1 1-e 1-e 0+e],[0 0 1 1-e 0+e 0+e],c2);patch([0 0 1 1-e 0+e 0+e],[0 1 1 1-e 1-e 0+e],c3);plot([0 1 1 0 0],[0 0 1 1 0]);disp('Weights');
  "IW{1,1}(19,:)'" : Constant  Value=[-0.69192820872236715512570981445605866611003875732421875;-1.0115896887588913255484612818690948188304901123046875;0.2082050329143752265270705947841634042561054229736328125;1.4276170938064451920723740840912796556949615478515625;0.60289644057316038594507290326873771846294403076171875;0.491245567452074427539088219418772496283054351806640625]
      mask Display: e = 0.06;c1 = [120 150 230]/255;c2 = ([120 150 230]+0)/383;c3 = ([120 150 230]+128)/383;patch([0 1 1 0],[0 0 1 1],c1);patch([0 1 1 1-e 1-e 0+e],[0 0 1 1-e 0+e 0+e],c2);patch([0 0 1 1-e 0+e 0+e],[0 1 1 1-e 1-e 0+e],c3);plot([0 1 1 0 0],[0 0 1 1 0]);disp('Weights');
  "IW{1,1}(2,:)'" : Constant  Value=[0.819069212007324409796638065017759799957275390625;1.4205841344905445478019601068808697164058685302734375;-0.2087539526108411480631588119649677537381649017333984375;0.5615055630163883204630792533862404525279998779296875;0.7621159660466625407337915021344088017940521240234375;-0.25482421381122211112568720636772923171520233154296875]
      mask Display: e = 0.06;c1 = [120 150 230]/255;c2 = ([120 150 230]+0)/383;c3 = ([120 150 230]+128)/383;patch([0 1 1 0],[0 0 1 1],c1);patch([0 1 1 1-e 1-e 0+e],[0 0 1 1-e 0+e 0+e],c2);patch([0 0 1 1-e 0+e 0+e],[0 1 1 1-e 1-e 0+e],c3);plot([0 1 1 0 0],[0 0 1 1 0]);disp('Weights');
  "IW{1,1}(20,:)'" : Constant  Value=[-1.223472713315403748168819220154546201229095458984375;1.02781452349469848428498153225518763065338134765625;-0.5016143513805861875454183973488397896289825439453125;-0.76512208370276379998387028535944409668445587158203125;-0.343872743653884926917640996180125512182712554931640625;-0.8302771328935032446594277644180692732334136962890625]
      mask Display: e = 0.06;c1 = [120 150 230]/255;c2 = ([120 150 230]+0)/383;c3 = ([120 150 230]+128)/383;patch([0 1 1 0],[0 0 1 1],c1);patch([0 1 1 1-e 1-e 0+e],[0 0 1 1-e 0+e 0+e],c2);patch([0 0 1 1-e 0+e 0+e],[0 1 1 1-e 1-e 0+e],c3);plot([0 1 1 0 0],[0 0 1 1 0]);disp('Weights');
  "IW{1,1}(21,:)'" : Constant  Value=[0.96329922717340188409451684492523781955242156982421875;-0.6551169661280218381449458320275880396366119384765625;-0.50582440032005393515390778702567331492900848388671875;0.046064824593341609226815336342042428441345691680908203125;1.406097969527585700433292004163376986980438232421875;-1.30481552967731406766915824846364557743072509765625]
      mask Display: e = 0.06;c1 = [120 150 230]/255;c2 = ([120 150 230]+0)/383;c3 = ([120 150 230]+128)/383;patch([0 1 1 0],[0 0 1 1],c1);patch([0 1 1 1-e 1-e 0+e],[0 0 1 1-e 0+e 0+e],c2);patch([0 0 1 1-e 0+e 0+e],[0 1 1 1-e 1-e 0+e],c3);plot([0 1 1 0 0],[0 0 1 1 0]);disp('Weights');
  "IW{1,1}(22,:)'" : Constant  Value=[1.2788674220914140189364616162492893636226654052734375;-0.499205108866402846867771359029575251042842864990234375;0.12542267272189933091652846997021697461605072021484375;-0.54779174719712830921025670249946415424346923828125;0.97010399881503683872097099083475768566131591796875;0.613862465609015917067381451488472521305084228515625]
      mask Display: e = 0.06;c1 = [120 150 230]/255;c2 = ([120 150 230]+0)/383;c3 = ([120 150 230]+128)/383;patch([0 1 1 0],[0 0 1 1],c1);patch([0 1 1 1-e 1-e 0+e],[0 0 1 1-e 0+e 0+e],c2);patch([0 0 1 1-e 0+e 0+e],[0 1 1 1-e 1-e 0+e],c3);plot([0 1 1 0 0],[0 0 1 1 0]);disp('Weights');
  "IW{1,1}(23,:)'" : Constant  Value=[2.1742358562138814903619277174584567546844482421875;0.7779663865511003972841308495844714343547821044921875;0.11376764528600201431540739349657087586820125579833984375;-0.321381834602109339726894177147187292575836181640625;0.31338586648281763213930162237375043332576751708984375;0.8184780163425291465983946181950159370899200439453125]
      mask Display: e = 0.06;c1 = [120 150 230]/255;c2 = ([120 150 230]+0)/383;c3 = ([120 150 230]+128)/383;patch([0 1 1 0],[0 0 1 1],c1);patch([0 1 1 1-e 1-e 0+e],[0 0 1 1-e 0+e 0+e],c2);patch([0 0 1 1-e 0+e 0+e],[0 1 1 1-e 1-e 0+e],c3);plot([0 1 1 0 0],[0 0 1 1 0]);disp('Weights');
  "IW{1,1}(24,:)'" : Constant  Value=[-0.920122625825073203742476835031993687152862548828125;1.7985903786357282374552823966951109468936920166015625;-0.449335796921472019338494874318712390959262847900390625;0.37211945524182443723049118489143438637256622314453125;-0.268179811625878616876406113078701309859752655029296875;-0.99187628535014782382717157815932296216487884521484375]
      mask Display: e = 0.06;c1 = [120 150 230]/255;c2 = ([120 150 230]+0)/383;c3 = ([120 150 230]+128)/383;patch([0 1 1 0],[0 0 1 1],c1);patch([0 1 1 1-e 1-e 0+e],[0 0 1 1-e 0+e 0+e],c2);patch([0 0 1 1-e 0+e 0+e],[0 1 1 1-e 1-e 0+e],c3);plot([0 1 1 0 0],[0 0 1 1 0]);disp('Weights');
  "IW{1,1}(25,:)'" : Constant  Value=[-0.7468657722437128665404770799796096980571746826171875;0.9514243031970905928318416044930927455425262451171875;-0.19912347847005718026736076353699900209903717041015625;0.42273079982580286095839028348564170300960540771484375;-0.454298439023558542348979472080827690660953521728515625;0.1158651407635991337219394381463644094765186309814453125]
      mask Display: e = 0.06;c1 = [120 150 230]/255;c2 = ([120 150 230]+0)/383;c3 = ([120 150 230]+128)/383;patch([0 1 1 0],[0 0 1 1],c1);patch([0 1 1 1-e 1-e 0+e],[0 0 1 1-e 0+e 0+e],c2);patch([0 0 1 1-e 0+e 0+e],[0 1 1 1-e 1-e 0+e],c3);plot([0 1 1 0 0],[0 0 1 1 0]);disp('Weights');
  "IW{1,1}(3,:)'" : Constant  Value=[0.52707559518076940729969237509067170321941375732421875;-1.35807461272378393601911739096976816654205322265625;0.6803855694700444711742193248937837779521942138671875;0.5457109471856937954470367913017980754375457763671875;-0.87266721000643909800231767803779803216457366943359375;0.354606028999767397547060454598977230489253997802734375]
      mask Display: e = 0.06;c1 = [120 150 230]/255;c2 = ([120 150 230]+0)/383;c3 = ([120 150 230]+128)/383;patch([0 1 1 0],[0 0 1 1],c1);patch([0 1 1 1-e 1-e 0+e],[0 0 1 1-e 0+e 0+e],c2);patch([0 0 1 1-e 0+e 0+e],[0 1 1 1-e 1-e 0+e],c3);plot([0 1 1 0 0],[0 0 1 1 0]);disp('Weights');
  "IW{1,1}(4,:)'" : Constant  Value=[0.5348763590344882690175154493772424757480621337890625;-2.94460120006832237748994884896092116832733154296875;0.25881394439468252688385518922586925327777862548828125;-0.988869737367270573713540215976536273956298828125;-1.34291304141692702245336477062664926052093505859375;0.8873294643855762497963723944849334657192230224609375]
      mask Display: e = 0.06;c1 = [120 150 230]/255;c2 = ([120 150 230]+0)/383;c3 = ([120 150 230]+128)/383;patch([0 1 1 0],[0 0 1 1],c1);patch([0 1 1 1-e 1-e 0+e],[0 0 1 1-e 0+e 0+e],c2);patch([0 0 1 1-e 0+e 0+e],[0 1 1 1-e 1-e 0+e],c3);plot([0 1 1 0 0],[0 0 1 1 0]);disp('Weights');
  "IW{1,1}(5,:)'" : Constant  Value=[-0.2409305267371661951614214558503590524196624755859375;1.3517602448933578873635497075156308710575103759765625;0.671714233157041373800666406168602406978607177734375;0.1699364545961201400370299552378128282725811004638671875;1.4733154643789483362326109272544272243976593017578125;0.44108263254802881903060551849193871021270751953125]
      mask Display: e = 0.06;c1 = [120 150 230]/255;c2 = ([120 150 230]+0)/383;c3 = ([120 150 230]+128)/383;patch([0 1 1 0],[0 0 1 1],c1);patch([0 1 1 1-e 1-e 0+e],[0 0 1 1-e 0+e 0+e],c2);patch([0 0 1 1-e 0+e 0+e],[0 1 1 1-e 1-e 0+e],c3);plot([0 1 1 0 0],[0 0 1 1 0]);disp('Weights');
  "IW{1,1}(6,:)'" : Constant  Value=[-0.29966099248417654710152646657661534845829010009765625;2.155080979873955637771132387570105493068695068359375;-0.5456468341177356240478957261075265705585479736328125;1.29078953244448957349277407047338783740997314453125;0.66091237151677351135958815575577318668365478515625;0.7268233797996483946946000287425704300403594970703125]
      mask Display: e = 0.06;c1 = [120 150 230]/255;c2 = ([120 150 230]+0)/383;c3 = ([120 150 230]+128)/383;patch([0 1 1 0],[0 0 1 1],c1);patch([0 1 1 1-e 1-e 0+e],[0 0 1 1-e 0+e 0+e],c2);patch([0 0 1 1-e 0+e 0+e],[0 1 1 1-e 1-e 0+e],c3);plot([0 1 1 0 0],[0 0 1 1 0]);disp('Weights');
  "IW{1,1}(7,:)'" : Constant  Value=[-0.5134442442948008444858487564488314092159271240234375;-0.046290477876960854641819054222651175223290920257568359375;-0.2734432707170408871633071612450294196605682373046875;-0.2045817861686594352210732949970406480133533477783203125;0.6178838573936122902097167752799578011035919189453125;0.8082262562382600545873856390244327485561370849609375]
      mask Display: e = 0.06;c1 = [120 150 230]/255;c2 = ([120 150 230]+0)/383;c3 = ([120 150 230]+128)/383;patch([0 1 1 0],[0 0 1 1],c1);patch([0 1 1 1-e 1-e 0+e],[0 0 1 1-e 0+e 0+e],c2);patch([0 0 1 1-e 0+e 0+e],[0 1 1 1-e 1-e 0+e],c3);plot([0 1 1 0 0],[0 0 1 1 0]);disp('Weights');
  "IW{1,1}(8,:)'" : Constant  Value=[0.350862775841264851184320150423445738852024078369140625;0.68910283718495712879104075909708626568317413330078125;0.401025938922157598742757045329199172556400299072265625;0.0211565590218434108893408307494610198773443698883056640625;-1.279037208798537772480585772427730262279510498046875;1.401791982737751851573193562217056751251220703125]
      mask Display: e = 0.06;c1 = [120 150 230]/255;c2 = ([120 150 230]+0)/383;c3 = ([120 150 230]+128)/383;patch([0 1 1 0],[0 0 1 1],c1);patch([0 1 1 1-e 1-e 0+e],[0 0 1 1-e 0+e 0+e],c2);patch([0 0 1 1-e 0+e 0+e],[0 1 1 1-e 1-e 0+e],c3);plot([0 1 1 0 0],[0 0 1 1 0]);disp('Weights');
  "IW{1,1}(9,:)'" : Constant  Value=[1.418233051281720946690256823785603046417236328125;-1.182436857788876860553273218101821839809417724609375;-0.96678645577470512240125799507950432598590850830078125;-0.1518551314846387223500556729050003923475742340087890625;-0.86831624417003328009201368331559933722019195556640625;-0.64704123302700822240041134136845357716083526611328125]
      mask Display: e = 0.06;c1 = [120 150 230]/255;c2 = ([120 150 230]+0)/383;c3 = ([120 150 230]+128)/383;patch([0 1 1 0],[0 0 1 1],c1);patch([0 1 1 1-e 1-e 0+e],[0 0 1 1-e 0+e 0+e],c2);patch([0 0 1 1-e 0+e 0+e],[0 1 1 1-e 1-e 0+e],c3);plot([0 1 1 0 0],[0 0 1 1 0]);disp('Weights');
  Mux : Mux  Inputs=25
      mask Display: e = 0.06;c1 = [120 150 230]/255;c2 = ([120 150 230]+0)/383;c3 = ([120 150 230]+128)/383;patch([0 1 1 0],[0 0 1 1],c1);patch([0 1 1 1-e 1-e 0+e],[0 0 1 1-e 0+e 0+e],c2);patch([0 0 1 1-e 0+e 0+e],[0 1 1 1-e 1-e 0+e],c3);plot([0 1 1 0 0],[0 0 1 1 0]);disp('Mux');
  dotprod{1..25} (25 alike) : neural/Weight Functions/dotprod
      settings: SourceProductName=MATLAB Runtime - Deep Learning Toolbox  SourceProductBaseCode=Missing
  "iz{1,1}" : Outport  VectorParamsAs1DForOutWhenUnconnected=off
      mask Display: e = 0.06;c1 = [120 230 180]/255;c2 = ([120 230 180]+0)/(256+128);c3 = ([120 230 180]+128)/(256+128);patch([0 1 1 0],[0 0 1 1],c1);patch([0 1 1 1-e 1-e 0+e],[0 0 1 1-e 0+e 0+e],c2);patch([0 0 1 1-e 0+e 0+e],[0 1 1 1-e 1-e 0+e],c3);plot([0 1 1 0 0],[0 0 1 1 0]);
  wires:
  "IW{1,1}(1,:)'"/1 -> dotprod1/1
  "pd{1,1}"/1 -> dotprod1/2, dotprod2/2, dotprod3/2, dotprod4/2, dotprod5/2, dotprod6/2, dotprod7/2, dotprod8/2, dotprod9/2, dotprod10/2, dotprod11/2, dotprod12/2, dotprod13/2, dotprod14/2, dotprod15/2, dotprod16/2, dotprod17/2, dotprod18/2, dotprod19/2, dotprod20/2, dotprod21/2, dotprod22/2, dotprod23/2, dotprod24/2, dotprod25/2
  dotprod1/1 -> Mux/1
  "IW{1,1}(2,:)'"/1 -> dotprod2/1
  dotprod2/1 -> Mux/2
  "IW{1,1}(3,:)'"/1 -> dotprod3/1
  dotprod3/1 -> Mux/3
  "IW{1,1}(4,:)'"/1 -> dotprod4/1
  dotprod4/1 -> Mux/4
  "IW{1,1}(5,:)'"/1 -> dotprod5/1
  dotprod5/1 -> Mux/5
  "IW{1,1}(6,:)'"/1 -> dotprod6/1
  dotprod6/1 -> Mux/6
  "IW{1,1}(7,:)'"/1 -> dotprod7/1
  dotprod7/1 -> Mux/7
  "IW{1,1}(8,:)'"/1 -> dotprod8/1
  dotprod8/1 -> Mux/8
  "IW{1,1}(9,:)'"/1 -> dotprod9/1
  dotprod9/1 -> Mux/9
  "IW{1,1}(10,:)'"/1 -> dotprod10/1
  dotprod10/1 -> Mux/10
  "IW{1,1}(11,:)'"/1 -> dotprod11/1
  dotprod11/1 -> Mux/11
  "IW{1,1}(12,:)'"/1 -> dotprod12/1
  dotprod12/1 -> Mux/12
  "IW{1,1}(13,:)'"/1 -> dotprod13/1
  dotprod13/1 -> Mux/13
  "IW{1,1}(14,:)'"/1 -> dotprod14/1
  dotprod14/1 -> Mux/14
  "IW{1,1}(15,:)'"/1 -> dotprod15/1
  dotprod15/1 -> Mux/15
  "IW{1,1}(16,:)'"/1 -> dotprod16/1
  dotprod16/1 -> Mux/16
  "IW{1,1}(17,:)'"/1 -> dotprod17/1
  dotprod17/1 -> Mux/17
  "IW{1,1}(18,:)'"/1 -> dotprod18/1
  dotprod18/1 -> Mux/18
  "IW{1,1}(19,:)'"/1 -> dotprod19/1
  dotprod19/1 -> Mux/19
  "IW{1,1}(20,:)'"/1 -> dotprod20/1
  dotprod20/1 -> Mux/20
  "IW{1,1}(21,:)'"/1 -> dotprod21/1
  dotprod21/1 -> Mux/21
  "IW{1,1}(22,:)'"/1 -> dotprod22/1
  dotprod22/1 -> Mux/22
  "IW{1,1}(23,:)'"/1 -> dotprod23/1
  dotprod23/1 -> Mux/23
  "IW{1,1}(24,:)'"/1 -> dotprod24/1
  dotprod24/1 -> Mux/24
  "IW{1,1}(25,:)'"/1 -> dotprod25/1
  dotprod25/1 -> Mux/25
  Mux/1 -> "iz{1,1}"/1

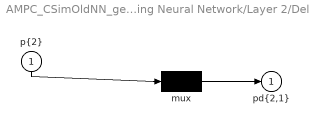
== system AMPC_CSimOldNN_genLinearModelBased/Subsystem/Function Fitting Neural Network/Layer 2/Delays 1 ==
  "p{2}" : Inport  PortDimensions=25
      mask Display: e = 0.06;c1 = [120 230 180]/255;c2 = ([120 230 180]+0)/(256+128);c3 = ([120 230 180]+128)/(256+128);patch([0 1 1 0],[0 0 1 1],c1);patch([0 1 1 1-e 1-e 0+e],[0 0 1 1-e 0+e 0+e],c2);patch([0 0 1 1-e 0+e 0+e],[0 1 1 1-e 1-e 0+e],c3);plot([0 1 1 0 0],[0 0 1 1 0]);
  mux : Mux  Inputs=1
      mask Display: e = 0.06;c1 = [120 150 230]/255;c2 = ([120 150 230]+0)/383;c3 = ([120 150 230]+128)/383;patch([0 1 1 0],[0 0 1 1],c1);patch([0 1 1 1-e 1-e 0+e],[0 0 1 1-e 0+e 0+e],c2);patch([0 0 1 1-e 0+e 0+e],[0 1 1 1-e 1-e 0+e],c3);plot([0 1 1 0 0],[0 0 1 1 0]);disp('Mux')
  "pd{2,1}" : Outport  VectorParamsAs1DForOutWhenUnconnected=off
      mask Display: e = 0.06;c1 = [120 230 180]/255;c2 = ([120 230 180]+0)/(256+128);c3 = ([120 230 180]+128)/(256+128);patch([0 1 1 0],[0 0 1 1],c1);patch([0 1 1 1-e 1-e 0+e],[0 0 1 1-e 0+e 0+e],c2);patch([0 0 1 1-e 0+e 0+e],[0 1 1 1-e 1-e 0+e],c3);plot([0 1 1 0 0],[0 0 1 1 0]);
  wires:
  "p{2}"/1 -> mux/1
  mux/1 -> "pd{2,1}"/1

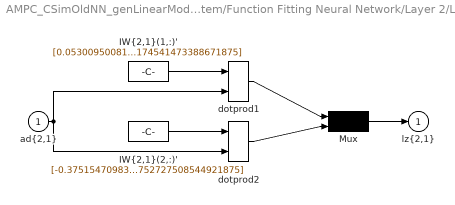
== system AMPC_CSimOldNN_genLinearModelBased/Subsystem/Function Fitting Neural Network/Layer 2/LW{2,1} ==
  "ad{2,1}" : Inport  PortDimensions=25
      mask Display: e = 0.06;c1 = [120 230 180]/255;c2 = ([120 230 180]+0)/(256+128);c3 = ([120 230 180]+128)/(256+128);patch([0 1 1 0],[0 0 1 1],c1);patch([0 1 1 1-e 1-e 0+e],[0 0 1 1-e 0+e 0+e],c2);patch([0 0 1 1-e 0+e 0+e],[0 1 1 1-e 1-e 0+e],c3);plot([0 1 1 0 0],[0 0 1 1 0]);
  "IW{2,1}(1,:)'" : Constant  Value=[0.053009500816631381636678810309604159556329250335693359375;1.068751779914871580245971927070058882236480712890625;0.8941755927975811868435584983672015368938446044921875;0.26666444265424960047283775566029362380504608154296875;1.9854215559896750686874611346866004168987274169921875;-0.061996390584446968430309965469859889708459377288818359375;-0.7599389840378567573253576483693905174732208251953125;-1.8953198972188689541695794105180539190769195556640625;1.27710150044223968990309003856964409351348876953125;1.0818234522679277542778208953677676618099212646484375;-1.9013012190243989696369908415363170206546783447265625;-1.4565290884924582126558334493893198668956756591796875;1.0871454996625884437122522285790182650089263916015625;1.18916750699715034755854503600858151912689208984375;-0.77329469543329254488384094656794331967830657958984375;-1.335247753105627932512788902386091649532318115234375;1.1370794018775078892957708376343362033367156982421875;0.292394494133218108000704660298652015626430511474609375;0.6910969489126503884079966155695728957653045654296875;1.5160004719763315872427256181254051625728607177734375;-1.3721078286370211873901325816405005753040313720703125;1.292941555738996495250603402382694184780120849609375;1.7138796645551959141329234626027755439281463623046875;-0.035139365064529477777899302282094140537083148956298828125;1.12598493238334196320238334010355174541473388671875]
      mask Display: e = 0.06;c1 = [120 150 230]/255;c2 = ([120 150 230]+0)/383;c3 = ([120 150 230]+128)/383;patch([0 1 1 0],[0 0 1 1],c1);patch([0 1 1 1-e 1-e 0+e],[0 0 1 1-e 0+e 0+e],c2);patch([0 0 1 1-e 0+e 0+e],[0 1 1 1-e 1-e 0+e],c3);plot([0 1 1 0 0],[0 0 1 1 0]);disp('weights');
  "IW{2,1}(2,:)'" : Constant  Value=[-0.3751547098353940068449219324975274503231048583984375;-0.91417283342699329207192704416229389607906341552734375;-0.17281979492504173645528453562292270362377166748046875;-1.107118138034655085988333667046390473842620849609375;0.1458148742536761466315198276788578368723392486572265625;0.8540653003652973751513854949735105037689208984375;0.2284368701578295690612918633632943965494632720947265625;0.1643582400806844756591118539290619082748889923095703125;-0.06650142004198549006144247641714173369109630584716796875;1.001777741426220558196291676722466945648193359375;-0.65315945190090285432660266451421193778514862060546875;-1.2713911175420176125072657669079490005970001220703125;1.3505144018127486216229726778692565858364105224609375;0.60722141728468159715959018285502679646015167236328125;-1.3227244308739709577338317103567533195018768310546875;1.0715503565368120764134118871879763901233673095703125;-0.53168100644631699491782228506053797900676727294921875;-0.96267136789897300719331951768253929913043975830078125;-0.29745905442390474515690357293351553380489349365234375;0.32415387176602428187521809377358295023441314697265625;0.496952388036444148156078881584107875823974609375;-0.0420948037311068834487315371006843633949756622314453125;0.99207643348153717877124790902598761022090911865234375;0.97866322498576197030928369713365100324153900146484375;0.86695627674721442712524321905220858752727508544921875]
      mask Display: e = 0.06;c1 = [120 150 230]/255;c2 = ([120 150 230]+0)/383;c3 = ([120 150 230]+128)/383;patch([0 1 1 0],[0 0 1 1],c1);patch([0 1 1 1-e 1-e 0+e],[0 0 1 1-e 0+e 0+e],c2);patch([0 0 1 1-e 0+e 0+e],[0 1 1 1-e 1-e 0+e],c3);plot([0 1 1 0 0],[0 0 1 1 0]);disp('weights');
  Mux : Mux  Inputs=2
      mask Display: e = 0.06;c1 = [120 150 230]/255;c2 = ([120 150 230]+0)/383;c3 = ([120 150 230]+128)/383;patch([0 1 1 0],[0 0 1 1],c1);patch([0 1 1 1-e 1-e 0+e],[0 0 1 1-e 0+e 0+e],c2);patch([0 0 1 1-e 0+e 0+e],[0 1 1 1-e 1-e 0+e],c3);plot([0 1 1 0 0],[0 0 1 1 0]);disp('Mux');
  dotprod1 : neural/Weight Functions/dotprod
      settings: SourceProductName=MATLAB Runtime - Deep Learning Toolbox  SourceProductBaseCode=Missing
  dotprod2 : neural/Weight Functions/dotprod
      settings: SourceProductName=MATLAB Runtime - Deep Learning Toolbox  SourceProductBaseCode=Missing
  "lz{2,1}" : Outport  VectorParamsAs1DForOutWhenUnconnected=off
      mask Display: e = 0.06;c1 = [120 230 180]/255;c2 = ([120 230 180]+0)/(256+128);c3 = ([120 230 180]+128)/(256+128);patch([0 1 1 0],[0 0 1 1],c1);patch([0 1 1 1-e 1-e 0+e],[0 0 1 1-e 0+e 0+e],c2);patch([0 0 1 1-e 0+e 0+e],[0 1 1 1-e 1-e 0+e],c3);plot([0 1 1 0 0],[0 0 1 1 0]);
  wires:
  "IW{2,1}(1,:)'"/1 -> dotprod1/1
  "ad{2,1}"/1 -> dotprod1/2, dotprod2/2
  dotprod1/1 -> Mux/1
  "IW{2,1}(2,:)'"/1 -> dotprod2/1
  dotprod2/1 -> Mux/2
  Mux/1 -> "lz{2,1}"/1

== matlab function AMPC_CSimOldNN_genLinearModelBased/Plant ==
  data: Vx input; Ac output; Cf input; Cr input; Bc output; Cc output; Dc output
function [Ac, Bc, Cc, Dc]  = fcn(Vx,Cf,Cr)

% Model parameters
m = 1650;
Iz = 3234;
lf = 1.4;
lr = 1.65;

% Continuous-time model
Ac=[-(Cf+Cr)/(m*Vx), -1-(lf*Cf-lr*Cr)/(m*Vx^2);
    -(lf*Cf-lr*Cr)/Iz, -(lf^2*Cf+lr^2*Cr)/(Iz*Vx)];

Bc=[Cf/(m*Vx);(lf*Cf)/Iz];

Cc=eye(2);

Dc=[0;0];

%dotX = Ac*x+Bc*steer;

== matlab function AMPC_CSimOldNN_genLinearModelBased/MATLAB Function1 ==
  data: Vx input; A output size=[2,2]; Cf input; Cr input; steer input; x input size=[2,1]; B output size=[2,1]; C output size=[2,2]; D output size=[2,1]; U output size=1; Y output size=[2,1]; X output size=[2,1]; DX output size=[2,1]
function [A,B,C,D,U,Y,X,DX] = fcn(Vx,Cf,Cr,steer,x)
% Sample time
Ts = 0.025;

% Model parameters
m = 1650;
Iz = 3234;
lf = 1.4;
lr = 1.65;

% Continuous-time model
Ac=[-(Cf+Cr)/(m*Vx), -1-(lf*Cf-lr*Cr)/(m*Vx^2);
    -(lf*Cf-lr*Cr)/Iz, -(lf^2*Cf+lr^2*Cr)/(Iz*Vx)];

Bc=[Cf/(m*Vx);(lf*Cf)/Iz];

Cc=eye(2);

Dc=zeros(2,1);

% Generate discrete-time model
nx = size(Ac,1);
nu = size(Bc,2);
M = expm([[Ac Bc]*Ts; zeros(nu,nx+nu)]);
A = M(1:nx,1:nx);
B = M(1:nx,nx+1:nx+nu);
C = Cc;
D = Dc;

% Nominal conditions for discrete-time plant
X = x;
U = steer;
Y = C*x + D*steer;
DX = A*x+B*steer-x;

== matlab function AMPC_CSimOldNN_genLinearModelBased/MATLAB Function2 ==
  data: beta input; out output; yawrate input
function out = fcn(beta,yawrate)

out=[beta;yawrate];
